simulink model "Taskspace_3R_SMC"  (R2015b)
settings: Solver=VariableStepAuto  StartTime=0.0  StopTime=20  MaxStep=0.0001  RelTol=1e-3
settings Model: Creator=hadi jooon  LastModifiedBy=hadi jooon

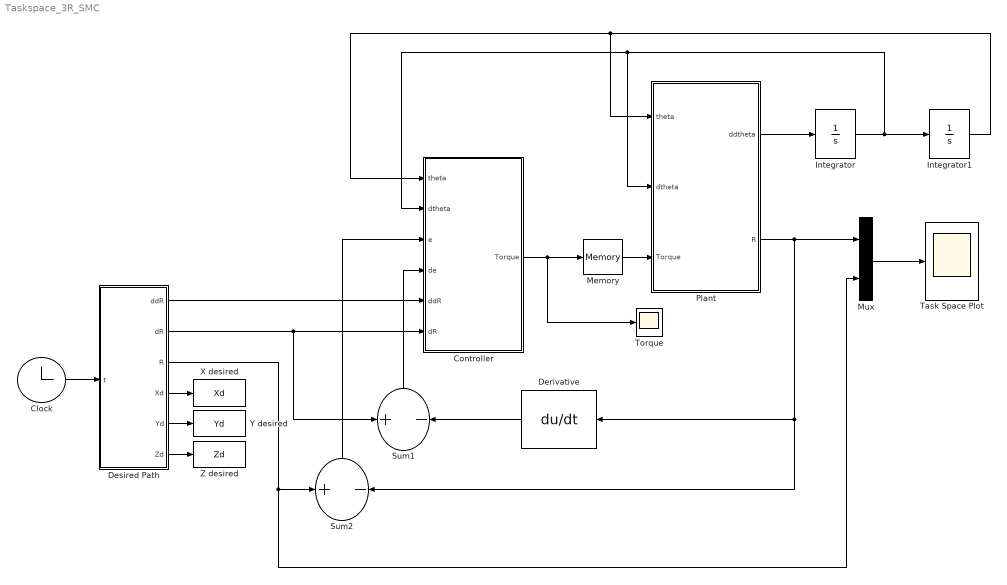
== system Taskspace_3R_SMC ==
  Clock : Clock
  Controller : MATLAB Function  TreatAsAtomicUnit=on
  Derivative : Derivative
  Desired Path : MATLAB Function  TreatAsAtomicUnit=on
  Integrator : Integrator  InitialCondition=zeros(3,1)
  Integrator1 : Integrator  InitialCondition=randn(3,1)
  Memory : Memory
  Mux : Mux  Inputs=2
  Plant : MATLAB Function  TreatAsAtomicUnit=on
  Sum1 : Sum  Inputs=+|-
  Sum2 : Sum  Inputs=+|-
  Task Space Plot : Scope
  Torque : Scope
  X desired : ToWorkspace  VariableName=Xd  SaveFormat=Timeseries  SampleTime=-1
  "Y desired " : ToWorkspace  VariableName=Yd  SaveFormat=Timeseries  SampleTime=-1
  "Z desired " : ToWorkspace  VariableName=Zd  SaveFormat=Timeseries  SampleTime=-1
  wires:
  Integrator/1 -> Integrator1/1, Controller/2(dtheta), Plant/2(dtheta)
  Integrator1/1 -> Plant/1(theta), Controller/1(theta)
  Plant/1(ddtheta) -> Integrator/1
  Controller/1(Torque) -> Torque/1, Memory/1
  Desired Path/1(ddR) -> Controller/5(ddR)
  Desired Path/3(R) -> Sum2/1, Mux/2
  Sum2/1 -> Controller/3(e)
  Desired Path/2(dR) -> Sum1/1, Controller/6(dR)
  Derivative/1 -> Sum1/2
  Sum1/1 -> Controller/4(de)
  Mux/1 -> Task Space Plot/1
  Clock/1 -> Desired Path/1(t)
  Memory/1 -> Plant/3(Torque)
  Desired Path/4(Xd) -> X desired/1
  Desired Path/5(Yd) -> "Y desired "/1
  Plant/2(R) -> Mux/1, Sum2/2, Derivative/1
  Desired Path/6(Zd) -> "Z desired "/1

== matlab function Taskspace_3R_SMC/Desired Path ==
  data: ddR output; dR output; t input; R output; Xd output; Yd output; Zd output
function [ddR , dR , R, Xd , Yd , Zd] = fcn(t)

    Xd = 2*(cos(t)+2);
    Yd = 2*(sin(t)+1);
    Zd = 6;

    dXd = -2*sin(t);
    dYd = 2*cos(t);
    dZd = 0;

    ddXd = -2*cos(t);
    ddYd = -2*sin(t);
    ddZd = 0;

    R = [Xd;Yd;Zd];
    dR = [dXd;dYd;dZd];
    ddR = [ddXd ; ddYd ;ddZd];

== matlab function Taskspace_3R_SMC/Plant ==
  data: ddtheta output; R output; theta input; dtheta input; Torque input
function [ddtheta, R]= fcn( theta , dtheta , Torque)
    
    m1 = 1; %kg
    m2 = 1 ; %kg
    m3 = 1 ; %kg

    L1 = 4 ; %m
    L2 = 4 ; %m
    L3 = 4 ; %m

    I1x = 1/12 * m1 * L1^2 ; %kg.N
    I2x = 1/12 * m2 * L2^2 ; %kg.N
    I3x = 1/12 * m3 * L3^2 ; %kg.N
    
    I1z = 1/3 * m1 * L1^2 ; %kg.N
    I2z = 1/3 * m2 * L2^2 ; %kg.N
    I3z = 1/3 * m3 * L3^2 ; %kg.N
    
    g = 9.8; % m/s^2
    
    t1 = theta(1);
    t2 = theta(2);
    t3 = theta(3);

    dt1 = dtheta(1);
    dt2 = dtheta(2);
    dt3 = dtheta(3);

    M = zeros(3,3) ;
   
    M(1,1) = I1z + I2z + I3z + (m2*((L2^2*cos(t1)^2*cos(t2)^2)/2 + (L2^2*cos(t2)^2*sin(t1)^2)/2))/2 + (m3*(2*cos(t1)^2*((L3*cos(t2 + t3))/2 + L2*cos(t2))^2 + 2*sin(t1)^2*((L3*cos(t2 + t3))/2 + L2*cos(t2))^2))/2; 
    M(1,2) = 0; 
    M(1,3) = 0; 
    M(2,1) = 0; 
    M(2,2) = I2x + I3x + (m2*((L2^2*cos(t2)^2)/2 + (L2^2*cos(t1)^2*sin(t2)^2)/2 + (L2^2*sin(t1)^2*sin(t2)^2)/2))/2 + (m3*(2*cos(t1)^2*((L3*sin(t2 + t3))/2 + L2*sin(t2))^2 + 2*sin(t1)^2*((L3*sin(t2 + t3))/2 + L2*sin(t2))^2 + 2*((L3*cos(t2 + t3))/2 + L2*cos(t2))^2))/2; 
    M(2,3) = I3x + (m3*(L3*cos(t2 + t3)*((L3*cos(t2 + t3))/2 + L2*cos(t2)) + L3*sin(t2 + t3)*sin(t1)^2*((L3*sin(t2 + t3))/2 + L2*sin(t2)) + L3*sin(t2 + t3)*cos(t1)^2*((L3*sin(t2 + t3))/2 + L2*sin(t2))))/2; 
    M(3,1) = 0; 
    M(3,2) = I3x + (m3*(L3*cos(t2 + t3)*((L3*cos(t2 + t3))/2 + L2*cos(t2)) + L3*sin(t2 + t3)*sin(t1)^2*((L3*sin(t2 + t3))/2 + L2*sin(t2)) + L3*sin(t2 + t3)*cos(t1)^2*((L3*sin(t2 + t3))/2 + L2*sin(t2))))/2; 
    M(3,3) = I3x + (m3*((L3^2*cos(t2 + t3)^2)/2 + (L3^2*sin(t2 + t3)^2*cos(t1)^2)/2 + (L3^2*sin(t2 + t3)^2*sin(t1)^2)/2))/2; 


    C = zeros(3,1);

    C(1,1) = - dt2*((m3*(2*cos(t1)*((L3*cos(t2 + t3))/2 + L2*cos(t2))*(dt2*sin(t1)*((L3*cos(t2 + t3))/2 + L2*cos(t2)) + dt1*cos(t1)*((L3*sin(t2 + t3))/2 + L2*sin(t2)) + (L3*dt3*cos(t2 + t3)*sin(t1))/2) - 2*sin(t1)*((L3*cos(t2 + t3))/2 + L2*cos(t2))*(dt2*cos(t1)*((L3*cos(t2 + t3))/2 + L2*cos(t2)) - dt1*sin(t1)*((L3*sin(t2 + t3))/2 + L2*sin(t2)) + (L3*dt3*cos(t2 + t3)*cos(t1))/2) + 2*sin(t1)*((L3*sin(t2 + t3))/2 + L2*sin(t2))*(dt1*sin(t1)*((L3*cos(t2 + t3))/2 + L2*cos(t2)) + dt2*cos(t1)*((L3*sin(t2 + t3))/2 + L2*sin(t2)) + (L3*dt3*sin(t2 + t3)*cos(t1))/2) - 2*cos(t1)*((L3*sin(t2 + t3))/2 + L2*sin(t2))*(dt2*sin(t1)*((L3*sin(t2 + t3))/2 + L2*sin(t2)) - dt1*cos(t1)*((L3*cos(t2 + t3))/2 + L2*cos(t2)) + (L3*dt3*sin(t2 + t3)*sin(t1))/2)))/2 + (m2*(L2*cos(t1)*cos(t2)*((L2*dt1*cos(t1)*sin(t2))/2 + (L2*dt2*cos(t2)*sin(t1))/2) + L2*cos(t1)*sin(t2)*((L2*dt1*cos(t1)*cos(t2))/2 - (L2*dt2*sin(t1)*sin(t2))/2) - L2*cos(t2)*sin(t1)*((L2*dt2*cos(t1)*cos(t2))/2 - (L2*dt1*sin(t1)*sin(t2))/2) + L2*sin(t1)*sin(t2)*((L2*dt1*cos(t2)*sin(t1))/2 + (L2*dt2*cos(t1)*sin(t2))/2)))/2) - (dt3*m3*(2*cos(t1)*((L3*cos(t2 + t3))/2 + L2*cos(t2))*((L3*dt1*sin(t2 + t3)*cos(t1))/2 + (L3*dt2*cos(t2 + t3)*sin(t1))/2 + (L3*dt3*cos(t2 + t3)*sin(t1))/2) - 2*sin(t1)*((L3*cos(t2 + t3))/2 + L2*cos(t2))*((L3*dt2*cos(t2 + t3)*cos(t1))/2 + (L3*dt3*cos(t2 + t3)*cos(t1))/2 - (L3*dt1*sin(t2 + t3)*sin(t1))/2) + L3*sin(t2 + t3)*sin(t1)*(dt1*sin(t1)*((L3*cos(t2 + t3))/2 + L2*cos(t2)) + dt2*cos(t1)*((L3*sin(t2 + t3))/2 + L2*sin(t2)) + (L3*dt3*sin(t2 + t3)*cos(t1))/2) - L3*sin(t2 + t3)*cos(t1)*(dt2*sin(t1)*((L3*sin(t2 + t3))/2 + L2*sin(t2)) - dt1*cos(t1)*((L3*cos(t2 + t3))/2 + L2*cos(t2)) + (L3*dt3*sin(t2 + t3)*sin(t1))/2)))/2;
    C(2,1) = g*(m3*((L3*cos(t2 + t3))/2 + L2*cos(t2)) + (L2*m2*cos(t2))/2) - (m3*(2*(dt2*cos(t1)*((L3*cos(t2 + t3))/2 + L2*cos(t2)) - dt1*sin(t1)*((L3*sin(t2 + t3))/2 + L2*sin(t2)) + (L3*dt3*cos(t2 + t3)*cos(t1))/2)*(dt1*sin(t1)*((L3*cos(t2 + t3))/2 + L2*cos(t2)) + dt2*cos(t1)*((L3*sin(t2 + t3))/2 + L2*sin(t2)) + (L3*dt3*sin(t2 + t3)*cos(t1))/2) + 2*(dt2*sin(t1)*((L3*cos(t2 + t3))/2 + L2*cos(t2)) + dt1*cos(t1)*((L3*sin(t2 + t3))/2 + L2*sin(t2)) + (L3*dt3*cos(t2 + t3)*sin(t1))/2)*(dt2*sin(t1)*((L3*sin(t2 + t3))/2 + L2*sin(t2)) - dt1*cos(t1)*((L3*cos(t2 + t3))/2 + L2*cos(t2)) + (L3*dt3*sin(t2 + t3)*sin(t1))/2) - 2*(dt2*((L3*cos(t2 + t3))/2 + L2*cos(t2)) + (L3*dt3*cos(t2 + t3))/2)*(dt2*((L3*sin(t2 + t3))/2 + L2*sin(t2)) + (L3*dt3*sin(t2 + t3))/2)))/2 + (m2*(2*((L2*dt1*cos(t1)*cos(t2))/2 - (L2*dt2*sin(t1)*sin(t2))/2)*((L2*dt1*cos(t1)*sin(t2))/2 + (L2*dt2*cos(t2)*sin(t1))/2) - 2*((L2*dt2*cos(t1)*cos(t2))/2 - (L2*dt1*sin(t1)*sin(t2))/2)*((L2*dt1*cos(t2)*sin(t1))/2 + (L2*dt2*cos(t1)*sin(t2))/2) + (L2^2*dt2^2*cos(t2)*sin(t2))/2))/2 + dt2*((m3*(2*cos(t1)*((L3*cos(t2 + t3))/2 + L2*cos(t2))*(dt1*sin(t1)*((L3*cos(t2 + t3))/2 + L2*cos(t2)) + dt2*cos(t1)*((L3*sin(t2 + t3))/2 + L2*sin(t2)) + (L3*dt3*sin(t2 + t3)*cos(t1))/2) - 2*((L3*cos(t2 + t3))/2 + L2*cos(t2))*(dt2*((L3*sin(t2 + t3))/2 + L2*sin(t2)) + (L3*dt3*sin(t2 + t3))/2) - 2*(dt2*((L3*cos(t2 + t3))/2 + L2*cos(t2)) + (L3*dt3*cos(t2 + t3))/2)*((L3*sin(t2 + t3))/2 + L2*sin(t2)) + 2*cos(t1)*((L3*sin(t2 + t3))/2 + L2*sin(t2))*(dt2*cos(t1)*((L3*cos(t2 + t3))/2 + L2*cos(t2)) - dt1*sin(t1)*((L3*sin(t2 + t3))/2 + L2*sin(t2)) + (L3*dt3*cos(t2 + t3)*cos(t1))/2) + 2*sin(t1)*((L3*cos(t2 + t3))/2 + L2*cos(t2))*(dt2*sin(t1)*((L3*sin(t2 + t3))/2 + L2*sin(t2)) - dt1*cos(t1)*((L3*cos(t2 + t3))/2 + L2*cos(t2)) + (L3*dt3*sin(t2 + t3)*sin(t1))/2) + 2*sin(t1)*((L3*sin(t2 + t3))/2 + L2*sin(t2))*(dt2*sin(t1)*((L3*cos(t2 + t3))/2 + L2*cos(t2)) + dt1*cos(t1)*((L3*sin(t2 + t3))/2 + L2*sin(t2)) + (L3*dt3*cos(t2 + t3)*sin(t1))/2)))/2 + (m2*(L2*cos(t1)*cos(t2)*((L2*dt1*cos(t2)*sin(t1))/2 + (L2*dt2*cos(t1)*sin(t2))/2) - L2^2*dt2*cos(t2)*sin(t2) + L2*cos(t1)*sin(t2)*((L2*dt2*cos(t1)*cos(t2))/2 - (L2*dt1*sin(t1)*sin(t2))/2) - L2*cos(t2)*sin(t1)*((L2*dt1*cos(t1)*cos(t2))/2 - (L2*dt2*sin(t1)*sin(t2))/2) + L2*sin(t1)*sin(t2)*((L2*dt1*cos(t1)*sin(t2))/2 + (L2*dt2*cos(t2)*sin(t1))/2)))/2) + (dt3*m3*(2*cos(t1)*((L3*sin(t2 + t3))/2 + L2*sin(t2))*((L3*dt2*cos(t2 + t3)*cos(t1))/2 + (L3*dt3*cos(t2 + t3)*cos(t1))/2 - (L3*dt1*sin(t2 + t3)*sin(t1))/2) - L3*sin(t2 + t3)*(dt2*((L3*cos(t2 + t3))/2 + L2*cos(t2)) + (L3*dt3*cos(t2 + t3))/2) - 2*((L3*cos(t2 + t3))/2 + L2*cos(t2))*((L3*dt2*sin(t2 + t3))/2 + (L3*dt3*sin(t2 + t3))/2) + 2*sin(t1)*((L3*sin(t2 + t3))/2 + L2*sin(t2))*((L3*dt1*sin(t2 + t3)*cos(t1))/2 + (L3*dt2*cos(t2 + t3)*sin(t1))/2 + (L3*dt3*cos(t2 + t3)*sin(t1))/2) + L3*cos(t2 + t3)*cos(t1)*(dt1*sin(t1)*((L3*cos(t2 + t3))/2 + L2*cos(t2)) + dt2*cos(t1)*((L3*sin(t2 + t3))/2 + L2*sin(t2)) + (L3*dt3*sin(t2 + t3)*cos(t1))/2) + L3*cos(t2 + t3)*sin(t1)*(dt2*sin(t1)*((L3*sin(t2 + t3))/2 + L2*sin(t2)) - dt1*cos(t1)*((L3*cos(t2 + t3))/2 + L2*cos(t2)) + (L3*dt3*sin(t2 + t3)*sin(t1))/2)))/2; 
    C(3,1) = (dt2*m3*(L3*cos(t2 + t3)*cos(t1)*(dt1*sin(t1)*((L3*cos(t2 + t3))/2 + L2*cos(t2)) + dt2*cos(t1)*((L3*sin(t2 + t3))/2 + L2*sin(t2)) + (L3*dt3*sin(t2 + t3)*cos(t1))/2) - L3*cos(t2 + t3)*(dt2*((L3*sin(t2 + t3))/2 + L2*sin(t2)) + (L3*dt3*sin(t2 + t3))/2) - L3*sin(t2 + t3)*(dt2*((L3*cos(t2 + t3))/2 + L2*cos(t2)) + (L3*dt3*cos(t2 + t3))/2) + L3*sin(t2 + t3)*cos(t1)*(dt2*cos(t1)*((L3*cos(t2 + t3))/2 + L2*cos(t2)) - dt1*sin(t1)*((L3*sin(t2 + t3))/2 + L2*sin(t2)) + (L3*dt3*cos(t2 + t3)*cos(t1))/2) + L3*sin(t2 + t3)*sin(t1)*(dt2*sin(t1)*((L3*cos(t2 + t3))/2 + L2*cos(t2)) + dt1*cos(t1)*((L3*sin(t2 + t3))/2 + L2*sin(t2)) + (L3*dt3*cos(t2 + t3)*sin(t1))/2) + L3*cos(t2 + t3)*sin(t1)*(dt2*sin(t1)*((L3*sin(t2 + t3))/2 + L2*sin(t2)) - dt1*cos(t1)*((L3*cos(t2 + t3))/2 + L2*cos(t2)) + (L3*dt3*sin(t2 + t3)*sin(t1))/2)))/2 - (m3*(2*((L3*dt2*cos(t2 + t3)*cos(t1))/2 + (L3*dt3*cos(t2 + t3)*cos(t1))/2 - (L3*dt1*sin(t2 + t3)*sin(t1))/2)*(dt1*sin(t1)*((L3*cos(t2 + t3))/2 + L2*cos(t2)) + dt2*cos(t1)*((L3*sin(t2 + t3))/2 + L2*sin(t2)) + (L3*dt3*sin(t2 + t3)*cos(t1))/2) - 2*(dt2*((L3*cos(t2 + t3))/2 + L2*cos(t2)) + (L3*dt3*cos(t2 + t3))/2)*((L3*dt2*sin(t2 + t3))/2 + (L3*dt3*sin(t2 + t3))/2) + 2*((L3*dt1*sin(t2 + t3)*cos(t1))/2 + (L3*dt2*cos(t2 + t3)*sin(t1))/2 + (L3*dt3*cos(t2 + t3)*sin(t1))/2)*(dt2*sin(t1)*((L3*sin(t2 + t3))/2 + L2*sin(t2)) - dt1*cos(t1)*((L3*cos(t2 + t3))/2 + L2*cos(t2)) + (L3*dt3*sin(t2 + t3)*sin(t1))/2)))/2 + (dt3*m3*(L3*cos(t2 + t3)*cos(t1)*(dt1*sin(t1)*((L3*cos(t2 + t3))/2 + L2*cos(t2)) + dt2*cos(t1)*((L3*sin(t2 + t3))/2 + L2*sin(t2)) + (L3*dt3*sin(t2 + t3)*cos(t1))/2) - L3*sin(t2 + t3)*(dt2*((L3*cos(t2 + t3))/2 + L2*cos(t2)) + (L3*dt3*cos(t2 + t3))/2) - L3*cos(t2 + t3)*((L3*dt2*sin(t2 + t3))/2 + (L3*dt3*sin(t2 + t3))/2) + L3*cos(t2 + t3)*sin(t1)*(dt2*sin(t1)*((L3*sin(t2 + t3))/2 + L2*sin(t2)) - dt1*cos(t1)*((L3*cos(t2 + t3))/2 + L2*cos(t2)) + (L3*dt3*sin(t2 + t3)*sin(t1))/2) + L3*sin(t2 + t3)*cos(t1)*((L3*dt2*cos(t2 + t3)*cos(t1))/2 + (L3*dt3*cos(t2 + t3)*cos(t1))/2 - (L3*dt1*sin(t2 + t3)*sin(t1))/2) + L3*sin(t2 + t3)*sin(t1)*((L3*dt1*sin(t2 + t3)*cos(t1))/2 + (L3*dt2*cos(t2 + t3)*sin(t1))/2 + (L3*dt3*cos(t2 + t3)*sin(t1))/2)))/2 + (L3*g*m3*cos(t2 + t3))/2; 


    ddtheta = M\( Torque -C) ;

    x0 = 0;
    y0 = 0;
    z0 = L1;

    x1 = cos(theta(1))*(L2 * cos(theta(2)));
    y1 = sin(theta(1))*( L2 * cos(theta(2)));
    z1 = L1+ L2 * sin( theta(2));

    x2 = cos(theta(1))*( L2 * cos(theta(2)) + L3 * cos(theta(2)+theta(3)) );
    y2 = sin(theta(1))*( L2 * cos(theta(2)) + L3 * cos(theta(2)+theta(3)) );
    z2 = L1+ L2 * sin( theta(2)) + L3 * sin(theta(2) + theta(3));

    X0 = [x0;y0;z0];
    X1 = [x1;y1;z1];
    R = [x2;y2;z2];

    J11 = -sin(theta(1))*(L2 * cos(theta(2)) + L3 * cos(theta(2) + theta(3)));
    J12 = -cos(theta(1))*(L2 * sin(theta(2)) + L3 * sin(theta(2) + theta(3)));
    J13 = -L3 * cos(theta(1))* sin(theta(2)+theta(3));

    J21 = cos(theta(1))*(L1 + L2 * cos(theta(2)) + L3 * cos(theta(2) + theta(3)));
    J22 = -sin(theta(1))*(L2 * sin(theta(2)) + L3 * sin(theta(2) + theta(3)));
    J23 =-L3 * sin(theta(1))* sin(theta(2)+theta(3));

    J31 = 0;
    J32 =  L2 * cos(theta(2)) + L3 * cos( theta(2) + theta(3));
    J33 =  L3 * cos( theta(2) + theta(3));

    J = [J11 J12 J13 ; J21 J22 J23 ; J31 J32 J33];

    dX = J * dtheta;

== matlab function Taskspace_3R_SMC/Controller ==
  data: theta input; dtheta input; e input; de input; Torque output; ddR input; dR input
function Torque = fcn(theta , dtheta , e , de , ddR , dR)
 
    
    m1 = 1; %kg
    m2 = 1 ; %kg
    m3 = 1 ; %kg

    L1 = 4 ; %m
    L2 = 4 ; %m
    L3 = 4 ; %m

    I1x = 1/12 * m1 * L1^2 ; %kg.N
    I2x = 1/12 * m2 * L2^2 ; %kg.N
    I3x = 1/12 * m3 * L3^2 ; %kg.N
    
    I1z = 1/3 * m1 * L1^2 ; %kg.N
    I2z = 1/3 * m2 * L2^2 ; %kg.N
    I3z = 1/3 * m3 * L3^2 ; %kg.N
    
    g = 9.8; % m/s^2
    
    t1 = theta(1);
    t2 = theta(2);
    t3 = theta(3);

    dt1 = dtheta(1);
    dt2 = dtheta(2);
    dt3 = dtheta(3);

    M = zeros(3,3) ;
   
    M(1,1) = I1z + I2z + I3z + (m2*((L2^2*cos(t1)^2*cos(t2)^2)/2 + (L2^2*cos(t2)^2*sin(t1)^2)/2))/2 + (m3*(2*cos(t1)^2*((L3*cos(t2 + t3))/2 + L2*cos(t2))^2 + 2*sin(t1)^2*((L3*cos(t2 + t3))/2 + L2*cos(t2))^2))/2; 
    M(1,2) = 0; 
    M(1,3) = 0; 
    M(2,1) = 0; 
    M(2,2) = I2x + I3x + (m2*((L2^2*cos(t2)^2)/2 + (L2^2*cos(t1)^2*sin(t2)^2)/2 + (L2^2*sin(t1)^2*sin(t2)^2)/2))/2 + (m3*(2*cos(t1)^2*((L3*sin(t2 + t3))/2 + L2*sin(t2))^2 + 2*sin(t1)^2*((L3*sin(t2 + t3))/2 + L2*sin(t2))^2 + 2*((L3*cos(t2 + t3))/2 + L2*cos(t2))^2))/2; 
    M(2,3) = I3x + (m3*(L3*cos(t2 + t3)*((L3*cos(t2 + t3))/2 + L2*cos(t2)) + L3*sin(t2 + t3)*sin(t1)^2*((L3*sin(t2 + t3))/2 + L2*sin(t2)) + L3*sin(t2 + t3)*cos(t1)^2*((L3*sin(t2 + t3))/2 + L2*sin(t2))))/2; 
    M(3,1) = 0; 
    M(3,2) = I3x + (m3*(L3*cos(t2 + t3)*((L3*cos(t2 + t3))/2 + L2*cos(t2)) + L3*sin(t2 + t3)*sin(t1)^2*((L3*sin(t2 + t3))/2 + L2*sin(t2)) + L3*sin(t2 + t3)*cos(t1)^2*((L3*sin(t2 + t3))/2 + L2*sin(t2))))/2; 
    M(3,3) = I3x + (m3*((L3^2*cos(t2 + t3)^2)/2 + (L3^2*sin(t2 + t3)^2*cos(t1)^2)/2 + (L3^2*sin(t2 + t3)^2*sin(t1)^2)/2))/2; 


    C = zeros(3,1);

    C(1,1) = - dt2*((m3*(2*cos(t1)*((L3*cos(t2 + t3))/2 + L2*cos(t2))*(dt2*sin(t1)*((L3*cos(t2 + t3))/2 + L2*cos(t2)) + dt1*cos(t1)*((L3*sin(t2 + t3))/2 + L2*sin(t2)) + (L3*dt3*cos(t2 + t3)*sin(t1))/2) - 2*sin(t1)*((L3*cos(t2 + t3))/2 + L2*cos(t2))*(dt2*cos(t1)*((L3*cos(t2 + t3))/2 + L2*cos(t2)) - dt1*sin(t1)*((L3*sin(t2 + t3))/2 + L2*sin(t2)) + (L3*dt3*cos(t2 + t3)*cos(t1))/2) + 2*sin(t1)*((L3*sin(t2 + t3))/2 + L2*sin(t2))*(dt1*sin(t1)*((L3*cos(t2 + t3))/2 + L2*cos(t2)) + dt2*cos(t1)*((L3*sin(t2 + t3))/2 + L2*sin(t2)) + (L3*dt3*sin(t2 + t3)*cos(t1))/2) - 2*cos(t1)*((L3*sin(t2 + t3))/2 + L2*sin(t2))*(dt2*sin(t1)*((L3*sin(t2 + t3))/2 + L2*sin(t2)) - dt1*cos(t1)*((L3*cos(t2 + t3))/2 + L2*cos(t2)) + (L3*dt3*sin(t2 + t3)*sin(t1))/2)))/2 + (m2*(L2*cos(t1)*cos(t2)*((L2*dt1*cos(t1)*sin(t2))/2 + (L2*dt2*cos(t2)*sin(t1))/2) + L2*cos(t1)*sin(t2)*((L2*dt1*cos(t1)*cos(t2))/2 - (L2*dt2*sin(t1)*sin(t2))/2) - L2*cos(t2)*sin(t1)*((L2*dt2*cos(t1)*cos(t2))/2 - (L2*dt1*sin(t1)*sin(t2))/2) + L2*sin(t1)*sin(t2)*((L2*dt1*cos(t2)*sin(t1))/2 + (L2*dt2*cos(t1)*sin(t2))/2)))/2) - (dt3*m3*(2*cos(t1)*((L3*cos(t2 + t3))/2 + L2*cos(t2))*((L3*dt1*sin(t2 + t3)*cos(t1))/2 + (L3*dt2*cos(t2 + t3)*sin(t1))/2 + (L3*dt3*cos(t2 + t3)*sin(t1))/2) - 2*sin(t1)*((L3*cos(t2 + t3))/2 + L2*cos(t2))*((L3*dt2*cos(t2 + t3)*cos(t1))/2 + (L3*dt3*cos(t2 + t3)*cos(t1))/2 - (L3*dt1*sin(t2 + t3)*sin(t1))/2) + L3*sin(t2 + t3)*sin(t1)*(dt1*sin(t1)*((L3*cos(t2 + t3))/2 + L2*cos(t2)) + dt2*cos(t1)*((L3*sin(t2 + t3))/2 + L2*sin(t2)) + (L3*dt3*sin(t2 + t3)*cos(t1))/2) - L3*sin(t2 + t3)*cos(t1)*(dt2*sin(t1)*((L3*sin(t2 + t3))/2 + L2*sin(t2)) - dt1*cos(t1)*((L3*cos(t2 + t3))/2 + L2*cos(t2)) + (L3*dt3*sin(t2 + t3)*sin(t1))/2)))/2;
    C(2,1) = g*(m3*((L3*cos(t2 + t3))/2 + L2*cos(t2)) + (L2*m2*cos(t2))/2) - (m3*(2*(dt2*cos(t1)*((L3*cos(t2 + t3))/2 + L2*cos(t2)) - dt1*sin(t1)*((L3*sin(t2 + t3))/2 + L2*sin(t2)) + (L3*dt3*cos(t2 + t3)*cos(t1))/2)*(dt1*sin(t1)*((L3*cos(t2 + t3))/2 + L2*cos(t2)) + dt2*cos(t1)*((L3*sin(t2 + t3))/2 + L2*sin(t2)) + (L3*dt3*sin(t2 + t3)*cos(t1))/2) + 2*(dt2*sin(t1)*((L3*cos(t2 + t3))/2 + L2*cos(t2)) + dt1*cos(t1)*((L3*sin(t2 + t3))/2 + L2*sin(t2)) + (L3*dt3*cos(t2 + t3)*sin(t1))/2)*(dt2*sin(t1)*((L3*sin(t2 + t3))/2 + L2*sin(t2)) - dt1*cos(t1)*((L3*cos(t2 + t3))/2 + L2*cos(t2)) + (L3*dt3*sin(t2 + t3)*sin(t1))/2) - 2*(dt2*((L3*cos(t2 + t3))/2 + L2*cos(t2)) + (L3*dt3*cos(t2 + t3))/2)*(dt2*((L3*sin(t2 + t3))/2 + L2*sin(t2)) + (L3*dt3*sin(t2 + t3))/2)))/2 + (m2*(2*((L2*dt1*cos(t1)*cos(t2))/2 - (L2*dt2*sin(t1)*sin(t2))/2)*((L2*dt1*cos(t1)*sin(t2))/2 + (L2*dt2*cos(t2)*sin(t1))/2) - 2*((L2*dt2*cos(t1)*cos(t2))/2 - (L2*dt1*sin(t1)*sin(t2))/2)*((L2*dt1*cos(t2)*sin(t1))/2 + (L2*dt2*cos(t1)*sin(t2))/2) + (L2^2*dt2^2*cos(t2)*sin(t2))/2))/2 + dt2*((m3*(2*cos(t1)*((L3*cos(t2 + t3))/2 + L2*cos(t2))*(dt1*sin(t1)*((L3*cos(t2 + t3))/2 + L2*cos(t2)) + dt2*cos(t1)*((L3*sin(t2 + t3))/2 + L2*sin(t2)) + (L3*dt3*sin(t2 + t3)*cos(t1))/2) - 2*((L3*cos(t2 + t3))/2 + L2*cos(t2))*(dt2*((L3*sin(t2 + t3))/2 + L2*sin(t2)) + (L3*dt3*sin(t2 + t3))/2) - 2*(dt2*((L3*cos(t2 + t3))/2 + L2*cos(t2)) + (L3*dt3*cos(t2 + t3))/2)*((L3*sin(t2 + t3))/2 + L2*sin(t2)) + 2*cos(t1)*((L3*sin(t2 + t3))/2 + L2*sin(t2))*(dt2*cos(t1)*((L3*cos(t2 + t3))/2 + L2*cos(t2)) - dt1*sin(t1)*((L3*sin(t2 + t3))/2 + L2*sin(t2)) + (L3*dt3*cos(t2 + t3)*cos(t1))/2) + 2*sin(t1)*((L3*cos(t2 + t3))/2 + L2*cos(t2))*(dt2*sin(t1)*((L3*sin(t2 + t3))/2 + L2*sin(t2)) - dt1*cos(t1)*((L3*cos(t2 + t3))/2 + L2*cos(t2)) + (L3*dt3*sin(t2 + t3)*sin(t1))/2) + 2*sin(t1)*((L3*sin(t2 + t3))/2 + L2*sin(t2))*(dt2*sin(t1)*((L3*cos(t2 + t3))/2 + L2*cos(t2)) + dt1*cos(t1)*((L3*sin(t2 + t3))/2 + L2*sin(t2)) + (L3*dt3*cos(t2 + t3)*sin(t1))/2)))/2 + (m2*(L2*cos(t1)*cos(t2)*((L2*dt1*cos(t2)*sin(t1))/2 + (L2*dt2*cos(t1)*sin(t2))/2) - L2^2*dt2*cos(t2)*sin(t2) + L2*cos(t1)*sin(t2)*((L2*dt2*cos(t1)*cos(t2))/2 - (L2*dt1*sin(t1)*sin(t2))/2) - L2*cos(t2)*sin(t1)*((L2*dt1*cos(t1)*cos(t2))/2 - (L2*dt2*sin(t1)*sin(t2))/2) + L2*sin(t1)*sin(t2)*((L2*dt1*cos(t1)*sin(t2))/2 + (L2*dt2*cos(t2)*sin(t1))/2)))/2) + (dt3*m3*(2*cos(t1)*((L3*sin(t2 + t3))/2 + L2*sin(t2))*((L3*dt2*cos(t2 + t3)*cos(t1))/2 + (L3*dt3*cos(t2 + t3)*cos(t1))/2 - (L3*dt1*sin(t2 + t3)*sin(t1))/2) - L3*sin(t2 + t3)*(dt2*((L3*cos(t2 + t3))/2 + L2*cos(t2)) + (L3*dt3*cos(t2 + t3))/2) - 2*((L3*cos(t2 + t3))/2 + L2*cos(t2))*((L3*dt2*sin(t2 + t3))/2 + (L3*dt3*sin(t2 + t3))/2) + 2*sin(t1)*((L3*sin(t2 + t3))/2 + L2*sin(t2))*((L3*dt1*sin(t2 + t3)*cos(t1))/2 + (L3*dt2*cos(t2 + t3)*sin(t1))/2 + (L3*dt3*cos(t2 + t3)*sin(t1))/2) + L3*cos(t2 + t3)*cos(t1)*(dt1*sin(t1)*((L3*cos(t2 + t3))/2 + L2*cos(t2)) + dt2*cos(t1)*((L3*sin(t2 + t3))/2 + L2*sin(t2)) + (L3*dt3*sin(t2 + t3)*cos(t1))/2) + L3*cos(t2 + t3)*sin(t1)*(dt2*sin(t1)*((L3*sin(t2 + t3))/2 + L2*sin(t2)) - dt1*cos(t1)*((L3*cos(t2 + t3))/2 + L2*cos(t2)) + (L3*dt3*sin(t2 + t3)*sin(t1))/2)))/2; 
    C(3,1) = (dt2*m3*(L3*cos(t2 + t3)*cos(t1)*(dt1*sin(t1)*((L3*cos(t2 + t3))/2 + L2*cos(t2)) + dt2*cos(t1)*((L3*sin(t2 + t3))/2 + L2*sin(t2)) + (L3*dt3*sin(t2 + t3)*cos(t1))/2) - L3*cos(t2 + t3)*(dt2*((L3*sin(t2 + t3))/2 + L2*sin(t2)) + (L3*dt3*sin(t2 + t3))/2) - L3*sin(t2 + t3)*(dt2*((L3*cos(t2 + t3))/2 + L2*cos(t2)) + (L3*dt3*cos(t2 + t3))/2) + L3*sin(t2 + t3)*cos(t1)*(dt2*cos(t1)*((L3*cos(t2 + t3))/2 + L2*cos(t2)) - dt1*sin(t1)*((L3*sin(t2 + t3))/2 + L2*sin(t2)) + (L3*dt3*cos(t2 + t3)*cos(t1))/2) + L3*sin(t2 + t3)*sin(t1)*(dt2*sin(t1)*((L3*cos(t2 + t3))/2 + L2*cos(t2)) + dt1*cos(t1)*((L3*sin(t2 + t3))/2 + L2*sin(t2)) + (L3*dt3*cos(t2 + t3)*sin(t1))/2) + L3*cos(t2 + t3)*sin(t1)*(dt2*sin(t1)*((L3*sin(t2 + t3))/2 + L2*sin(t2)) - dt1*cos(t1)*((L3*cos(t2 + t3))/2 + L2*cos(t2)) + (L3*dt3*sin(t2 + t3)*sin(t1))/2)))/2 - (m3*(2*((L3*dt2*cos(t2 + t3)*cos(t1))/2 + (L3*dt3*cos(t2 + t3)*cos(t1))/2 - (L3*dt1*sin(t2 + t3)*sin(t1))/2)*(dt1*sin(t1)*((L3*cos(t2 + t3))/2 + L2*cos(t2)) + dt2*cos(t1)*((L3*sin(t2 + t3))/2 + L2*sin(t2)) + (L3*dt3*sin(t2 + t3)*cos(t1))/2) - 2*(dt2*((L3*cos(t2 + t3))/2 + L2*cos(t2)) + (L3*dt3*cos(t2 + t3))/2)*((L3*dt2*sin(t2 + t3))/2 + (L3*dt3*sin(t2 + t3))/2) + 2*((L3*dt1*sin(t2 + t3)*cos(t1))/2 + (L3*dt2*cos(t2 + t3)*sin(t1))/2 + (L3*dt3*cos(t2 + t3)*sin(t1))/2)*(dt2*sin(t1)*((L3*sin(t2 + t3))/2 + L2*sin(t2)) - dt1*cos(t1)*((L3*cos(t2 + t3))/2 + L2*cos(t2)) + (L3*dt3*sin(t2 + t3)*sin(t1))/2)))/2 + (dt3*m3*(L3*cos(t2 + t3)*cos(t1)*(dt1*sin(t1)*((L3*cos(t2 + t3))/2 + L2*cos(t2)) + dt2*cos(t1)*((L3*sin(t2 + t3))/2 + L2*sin(t2)) + (L3*dt3*sin(t2 + t3)*cos(t1))/2) - L3*sin(t2 + t3)*(dt2*((L3*cos(t2 + t3))/2 + L2*cos(t2)) + (L3*dt3*cos(t2 + t3))/2) - L3*cos(t2 + t3)*((L3*dt2*sin(t2 + t3))/2 + (L3*dt3*sin(t2 + t3))/2) + L3*cos(t2 + t3)*sin(t1)*(dt2*sin(t1)*((L3*sin(t2 + t3))/2 + L2*sin(t2)) - dt1*cos(t1)*((L3*cos(t2 + t3))/2 + L2*cos(t2)) + (L3*dt3*sin(t2 + t3)*sin(t1))/2) + L3*sin(t2 + t3)*cos(t1)*((L3*dt2*cos(t2 + t3)*cos(t1))/2 + (L3*dt3*cos(t2 + t3)*cos(t1))/2 - (L3*dt1*sin(t2 + t3)*sin(t1))/2) + L3*sin(t2 + t3)*sin(t1)*((L3*dt1*sin(t2 + t3)*cos(t1))/2 + (L3*dt2*cos(t2 + t3)*sin(t1))/2 + (L3*dt3*cos(t2 + t3)*sin(t1))/2)))/2 + (L3*g*m3*cos(t2 + t3))/2; 


    J = zeros(3,3);

    J(1,1) = -sin(t1)*(L3*cos(t2 + t3) + L2*cos(t2)); 
    J(1,2) = -cos(t1)*(L3*sin(t2 + t3) + L2*sin(t2)); 
    J(1,3) = -L3*sin(t2 + t3)*cos(t1); 
    J(2,1) = cos(t1)*(L3*cos(t2 + t3) + L2*cos(t2)); 
    J(2,2) = -sin(t1)*(L3*sin(t2 + t3) + L2*sin(t2)); 
    J(2,3) = -L3*sin(t2 + t3)*sin(t1); 
    J(3,1) = 0; 
    J(3,2) = L3*cos(t2 + t3) + L2*cos(t2); 
    J(3,3) = L3*cos(t2 + t3); 

    dJ = zeros(3,3);

    dJ(1,1) = dt2*sin(t1)*(L3*sin(t2 + t3) + L2*sin(t2)) - dt1*cos(t1)*(L3*cos(t2 + t3) + L2*cos(t2)) + L3*dt3*sin(t2 + t3)*sin(t1); 
    dJ(1,2) = dt1*sin(t1)*(L3*sin(t2 + t3) + L2*sin(t2)) - dt2*cos(t1)*(L3*cos(t2 + t3) + L2*cos(t2)) - L3*dt3*cos(t2 + t3)*cos(t1); 
    dJ(1,3) = L3*dt1*sin(t2 + t3)*sin(t1) - L3*dt3*cos(t2 + t3)*cos(t1) - L3*dt2*cos(t2 + t3)*cos(t1); 
    dJ(2,1) = - dt1*sin(t1)*(L3*cos(t2 + t3) + L2*cos(t2)) - dt2*cos(t1)*(L3*sin(t2 + t3) + L2*sin(t2)) - L3*dt3*sin(t2 + t3)*cos(t1); 
    dJ(2,2) = - dt2*sin(t1)*(L3*cos(t2 + t3) + L2*cos(t2)) - dt1*cos(t1)*(L3*sin(t2 + t3) + L2*sin(t2)) - L3*dt3*cos(t2 + t3)*sin(t1); 
    dJ(2,3) = - L3*dt1*sin(t2 + t3)*cos(t1) - L3*dt2*cos(t2 + t3)*sin(t1) - L3*dt3*cos(t2 + t3)*sin(t1); 
    dJ(3,1) = 0; 
    dJ(3,2) = - dt2*(L3*sin(t2 + t3) + L2*sin(t2)) - L3*dt3*sin(t2 + t3); 
    dJ(3,3) = - L3*dt2*sin(t2 + t3) - L3*dt3*sin(t2 + t3); 


    lamda = 10 * eye(3);
    k1  = 10 * eye(3);

    s = de + lamda * e  ;

    ddq = J\(ddR + lamda * de - dJ * dtheta + k1* atan(s/0.05) );
    
    Torque = C  + (M * ddq);
